simulink model "homework1_2"  (R2023a)
settings: Solver=VariableStepAuto  StartTime=0.0  StopTime=4  RelTol=1e-3
libraries: spsThyristorLib x4, spsVoltageMeasurementLib x3, spsACVoltageSourceLib x1, spsCurrentMeasurementLib x1, spsLinearTransformerLib x1, spsSeriesRLCBranchLib x1, sps_lib x1
settings Model: Creator=zou20  LastModifiedBy=zou20

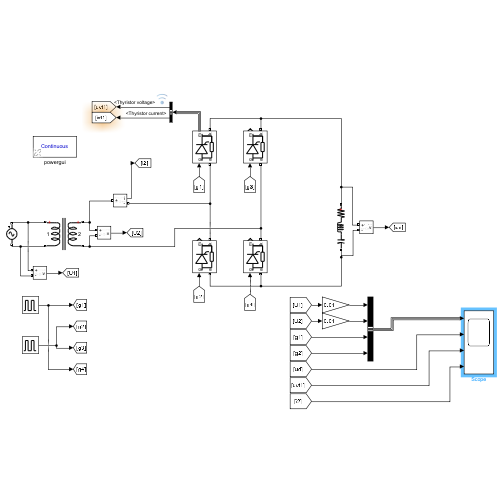
[thumbnail: Simulink's stored preview of the top-level diagram]
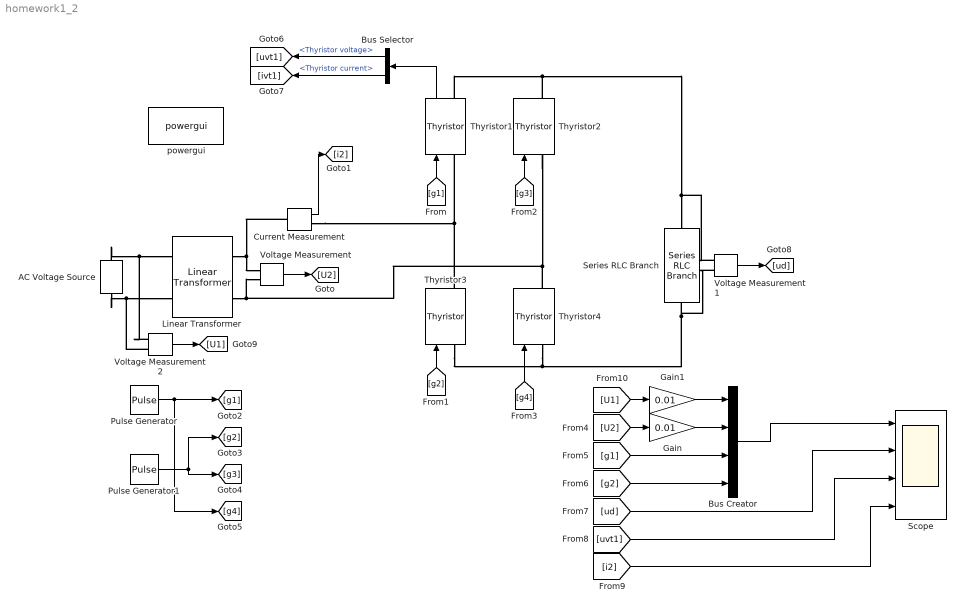
== system homework1_2 ==
  AC Voltage Source : spsACVoltageSourceLib/AC Voltage Source  Amplitude=311  Phase=0  Frequency=50  SampleTime=0  Measurements=None  BusType=swing  Pref=10e3  Qref=0  Qmin=-inf  Qmax=+inf
  Bus Creator : BusCreator  Inputs=4
  Bus Selector : BusSelector  OutputSignals=Thyristor voltage,Thyristor current
  Current Measurement : spsCurrentMeasurementLib/Current Measurement  PhasorSimulation=off  OutputType=Complex  PSBequivalent=0
  Gain : Gain  Gain=0.01
  Gain1 : Gain  Gain=0.01
  Linear Transformer : spsLinearTransformerLib/Linear Transformer  UNITS=pu  NominalPower=[ 10e3 50 ]  winding1="[ 220  0  0 ]"  winding2="[ 110  0  0 ]"  ThreeWindings=off  winding3=[ 315e3 0.002 0.08 ]  RmLm=[ inf inf ]  Measurements=None  DataType=off
  Pulse Generator : DiscretePulseGenerator  PulseType=Time based  Amplitude=3  Period=0.02  PulseWidth=10  PhaseDelay=0.02/360*30
  Pulse Generator1 : DiscretePulseGenerator  PulseType=Time based  Amplitude=3  Period=0.02  PulseWidth=10  PhaseDelay=0.01+0.02/360*30
  Scope : Scope  NumInputPorts=4
  Series RLC Branch : spsSeriesRLCBranchLib/Series RLC Branch  LConnTagsString=__new0  RConnTagsString=__new0  BranchType=RLC  Resistance=1000  Inductance=0  SetiL0=off  InitialCurrent=0  Capacitance=0  Setx0=off  InitialVoltage=0  Measurements=None
  Thyristor1 : spsThyristorLib/Thyristor  Ron=0.001  Lon=0  Vf=0.8  IC=0  Rs=1e5  Cs=inf  Measurements=on
  Thyristor2 : spsThyristorLib/Thyristor  Ron=0.001  Lon=0  Vf=0.8  IC=0  Rs=500  Cs=250e-9  Measurements=on
  Thyristor3 : spsThyristorLib/Thyristor  Ron=0.001  Lon=0  Vf=0.8  IC=0  Rs=500  Cs=250e-9  Measurements=on
  Thyristor4 : spsThyristorLib/Thyristor  Ron=0.001  Lon=0  Vf=0.8  IC=0  Rs=500  Cs=250e-9  Measurements=on
  Voltage Measurement : spsVoltageMeasurementLib/Voltage Measurement  PhasorSimulation=off  OutputType=Complex  PSBequivalent=0
  Voltage Measurement1 : spsVoltageMeasurementLib/Voltage Measurement  PhasorSimulation=off  OutputType=Complex  PSBequivalent=0
  Voltage Measurement2 : spsVoltageMeasurementLib/Voltage Measurement  PhasorSimulation=off  OutputType=Complex  PSBequivalent=0
  powergui : sps_lib/powergui  Priority=1  SimulationMode=Continuous  SampleTime=50e-6  frequency=60  Iterations=50  frequencyindice=50  Pbase=100e6  ErrMax=1e-4  UnitsV=kV  UnitsW=MW  buscounter=0  FunctionMessages=off  echomessages=off  EnableUseOfTLC=off  CurrentSourceSwitches=off  DisableSnubberDevices=off  DisableRonSwitches=off  DisableVfSwitches=off  DisplayEquations=off  AutomaticDiscreteSolvers=off  SolverType=Tustin/Backward Euler (TBE)  Interpol=off  ExternalGateDelay=off  methode=off  Ts=100  x0status=blocks  SPID=on  SwTol=0  HookPort=off  NonlinearTolerance=1e-4  nMaxIteration=100  ContinueOnMaxIteration=off  RestoreLinks=warning  ResistiveCurrentMeasurement=off  Frange=[0:2:500]  Ylog=off  Xlog=on  ShowGrid=off  save=off  variable=ZData  structure=0  ZoomFFT=off  StartTime=0.0  cycles=1  DisplayStyle=1  fundamental=60  FreqAxis=off  MaxFrequency=1000  frequencyindicesteady=1  RmsSteady=1  display=off
  wires:
  Voltage Measurement/1 -> [U2]
  Current Measurement/1 -> [i2]
  Pulse Generator/1 -> [g4], [g1]
  [g1] -> Thyristor1/1
  Pulse Generator1/1 -> [g2], [g3]
  [g2] -> Thyristor3/1
  [g3] -> Thyristor2/1
  [g4] -> Thyristor4/1
  Thyristor1/1 -> Bus Selector/1
  Bus Selector/1 -> [uvt1]  "<Thyristor voltage>"
  Bus Selector/2 -> [ivt1]  "<Thyristor current>"
  Voltage Measurement1/1 -> [ud]
  [U2] -> Gain/1
  Gain/1 -> Bus Creator/2
  [g1] -> Bus Creator/3
  [g2] -> Bus Creator/4
  Bus Creator/1 -> Scope/1
  [ud] -> Scope/2
  [uvt1] -> Scope/3
  [i2] -> Scope/4
  Voltage Measurement2/1 -> [U1]
  [U1] -> Gain1/1
  Gain1/1 -> Bus Creator/1
  connections:
  AC Voltage Source/RConn1 -- Voltage Measurement2/LConn1 -- Linear Transformer/LConn1
  AC Voltage Source/LConn1 -- Voltage Measurement2/LConn2 -- Linear Transformer/LConn2
  Linear Transformer/RConn1 -- Current Measurement/LConn1 -- Voltage Measurement/LConn1
  Linear Transformer/RConn2 -- Thyristor4/RConn1 -- Thyristor2/LConn1 -- Voltage Measurement/LConn2
  Current Measurement/RConn1 -- Thyristor3/RConn1 -- Thyristor1/LConn1
  Thyristor1/RConn1 -- Thyristor2/RConn1 -- Voltage Measurement1/LConn1 -- Series RLC Branch/LConn1
  Thyristor3/LConn1 -- Thyristor4/LConn1 -- Voltage Measurement1/LConn2 -- Series RLC Branch/RConn1
